simulink model "Simple_drive_model_current"  (R2017b)
settings: Solver=VariableStepAuto  StartTime=0.0  StopTime=5  RelTol=1e-3  EnableMultiTasking=on
values from neighbouring files (symbols this model uses):
  i = 120    [Drive_simple_variables.m]
  Jload = 5    [Drive_simple_variables.m]
  Jmotor = Jgear + Jrot    (= 0.003335)    [Drive_simple_variables.m]
  Kcur_Fdb = round(Uadc_inp*kadc/Imax)    [Drive_simple_variables.m]
  kcur_i = 1/Te    (= 139.830508475)    [Drive_simple_variables.m]
  kcur_p = Wcutoff_c*Te*Rrot/(Kpwc*Kcur_Fdb)    [Drive_simple_variables.m]
  Ke = Km    (= 1.41666666667)    [Drive_simple_variables.m]
  Km = Mrate/I    (= 1.41666666667)    [Drive_simple_variables.m]
  Kpos_Fdb = kps_int    (= 63661.9772368)    [Drive_simple_variables.m]
  kpos_p = Wcutoff_pos*Ts    [Drive_simple_variables.m]
  Kpwc = Un/Uc    (= 45)    [Drive_simple_variables.m]
  Kspd_Fdb = kps_int*Ts    (= 63.6619772368)    [Drive_simple_variables.m]
  kspd_i = 1/Tspd    [Drive_simple_variables.m]
  kspd_p = Wcutoff_s/ksn    [Drive_simple_variables.m]
  Lrot = 0.0059    [Drive_simple_variables.m]
  Rrot = 0.8250    (= 0.825)    [Drive_simple_variables.m]
  Tpwc = 0.00014    [Drive_simple_variables.m]
  Ts = 1e-3    (= 0.001)    [Drive_simple_variables.m]
undefined symbols (not defined in the file or in its folder): Ampl, Wsr
settings Model: Creator=Руслан  LastModifiedBy=Ruslan
settings OptimizationCC: LifeSpan=inf
settings DebuggingCC: SFUnexpectedBacktrackingDiag=warning  SFNoUnconditionalDefaultTransitionDiag=warning  SFExecutionAtInitializationDiag=none
settings CodeAppCC: StateflowObjectComments=on
settings GRTTargetCC: TargetLangStandard=C89/C90 (ANSI)  GeneratePreprocessorConditionals=Disable all
settings ConfigComp: CovMetricSettings=dw  CovHtmlReporting=on  CovSaveCumulativeToWorkspaceVar=on  CovSaveSingleToWorkspaceVar=on  CovExternalEMLEnable=off

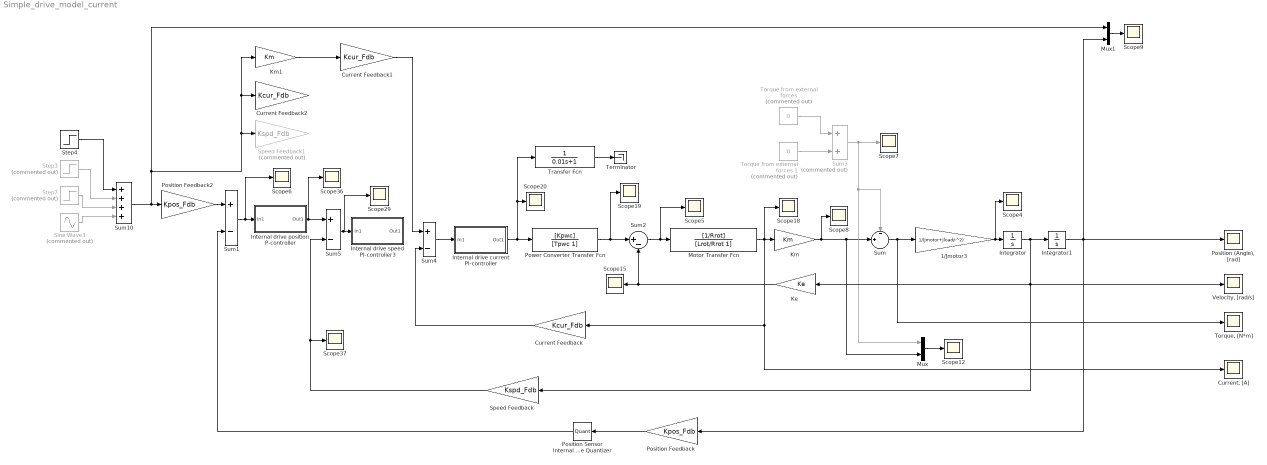
== system Simple_drive_model_current ==
  1/Jmotor3 : Gain  Gain=1/(Jmotor+Jload/i^2)  OutDataTypeStr=Inherit: Same as input  ParamDataTypeStr=Inherit: Same as input
  Current Feedback : Gain  Gain=Kcur_Fdb  OutDataTypeStr=Inherit: Same as input  ParamDataTypeStr=Inherit: Same as input
  Current Feedback1 : Gain  Gain=Kcur_Fdb  OutDataTypeStr=Inherit: Same as input  ParamDataTypeStr=Inherit: Same as input
  Current Feedback2 : Gain  Gain=Kcur_Fdb  OutDataTypeStr=Inherit: Same as input  ParamDataTypeStr=Inherit: Same as input
  "Current, [A]" : Scope
  Integrator : Integrator
  Integrator1 : Integrator
  Internal drive current PI-controller : Subsystem
  Internal drive position P-controller : Subsystem
  Internal drive speed PI-controller3 : Subsystem
  Ke : Gain  Gain=Ke  OutDataTypeStr=Inherit: Same as input  ParamDataTypeStr=Inherit: Same as input
  Km : Gain  Gain=Km  OutDataTypeStr=Inherit: Same as input  ParamDataTypeStr=Inherit: Same as input
  Km1 : Gain  Gain=Km  OutDataTypeStr=Inherit: Same as input  ParamDataTypeStr=Inherit: Same as input
  Motor Transfer Fcn : TransferFcn  Numerator=[1/Rrot]  Denominator=[Lrot/Rrot 1]
  Mux : Mux  Inputs=2
  Mux1 : Mux  Inputs=2
  "Position (Angle), [rad]" : Scope
  Position Feedback : Gain  Gain=Kpos_Fdb  OutDataTypeStr=Inherit: Same as input  ParamDataTypeStr=Inherit: Same as input
  Position Feedback2 : Gain  Gain=Kpos_Fdb  OutDataTypeStr=Inherit: Same as input  ParamDataTypeStr=Inherit: Same as input
  Position Sensor Internal Drive Quantizer : Quantizer  QuantizationInterval=1/Kpos_Fdb
  Power Converter Transfer Fcn : TransferFcn  Numerator=[Kpwc]  Denominator=[Tpwc 1]
  Scope{4..9,12,15,18..20,29,36..37} (14 alike) : Scope
  Sine Wave3 : Sin  Commented=on  Amplitude=Ampl  Frequency=Wsr  SampleTime=0
  Speed Feedback : Gain  Gain=Kspd_Fdb  OutDataTypeStr=Inherit: Same as input  ParamDataTypeStr=Inherit: Same as input
  Speed Feedback1 : Gain  Commented=on  Gain=Kspd_Fdb  OutDataTypeStr=Inherit: Same as input  ParamDataTypeStr=Inherit: Same as input
  Step3 : Step  Commented=on  Time=2  After=-1  SampleTime=0
  Step4 : Step  Time=0  SampleTime=0
  Step7 : Step  Commented=on  Time=2  SampleTime=0
  Sum : Sum  Inputs=-|+||
  Sum1 : Sum  Inputs=+-
  Sum10 : Sum  Inputs=4
  Sum2 : Sum  Inputs=|+-
  Sum3 : Sum  Commented=on  Inputs=2
  Sum4 : Sum  Inputs=+-
  Sum5 : Sum  Inputs=+-
  Terminator : Terminator
  "Torque from external forces " : Constant  Commented=on  Value=0
  Torque from external forces 1 : Constant  Commented=on  Value=0
  "Torque, [N*m]" : Scope
  Transfer Fcn : TransferFcn  Denominator=[0.01 1]
  "Velocity, [rad/s]" : Scope
  wires:
  Position Feedback/1 -> Position Sensor Internal Drive Quantizer/1
  Integrator1/1 -> Position Feedback/1, Mux1/2, "Position (Angle), [rad]"/1
  Sum4/1 -> Internal drive current PI-controller/1(In1)
  Sum5/1 -> Internal drive speed PI-controller3/1(In1), Scope29/1
  Speed Feedback/1 -> Scope37/1, Sum5/2
  Current Feedback/1 -> Sum4/2
  Sum1/1 -> Scope6/1, Internal drive position P-controller/1(In1)
  Km/1 -> Mux/2, Sum/2, Scope8/1
  Mux/1 -> Scope12/1
  Internal drive current PI-controller/1(Out1) -> Power Converter Transfer Fcn/1, Transfer Fcn/1, Scope20/1
  Power Converter Transfer Fcn/1 -> Scope19/1, Sum2/1
  Sum2/1 -> Scope5/1, Motor Transfer Fcn/1
  Sum/1 -> 1/Jmotor3/1, "Torque, [N*m]"/1
  1/Jmotor3/1 -> Scope4/1, Integrator/1
  Sum3/1 -> Sum/1, Mux/1, Scope7/1
  Motor Transfer Fcn/1 -> Km/1, Scope18/1, Current Feedback/1, "Current, [A]"/1
  Integrator/1 -> Integrator1/1, Speed Feedback/1, "Velocity, [rad/s]"/1, Ke/1
  Transfer Fcn/1 -> Terminator/1
  Step4/1 -> Sum10/1
  Step3/1 -> Sum10/2
  Step7/1 -> Sum10/3
  Position Feedback2/1 -> Sum1/1
  Mux1/1 -> Scope9/1
  Sum10/1 -> Position Feedback2/1, Mux1/1, Km1/1, Current Feedback2/1, Speed Feedback1/1
  Sine Wave3/1 -> Sum10/4
  Ke/1 -> Sum2/2, Scope15/1
  Position Sensor Internal Drive Quantizer/1 -> Sum1/2
  Internal drive position P-controller/1(Out1) -> Sum5/1, Scope36/1
  "Torque from external forces "/1 -> Sum3/1
  Torque from external forces 1/1 -> Sum3/2
  Km1/1 -> Current Feedback1/1
  Current Feedback1/1 -> Sum4/1

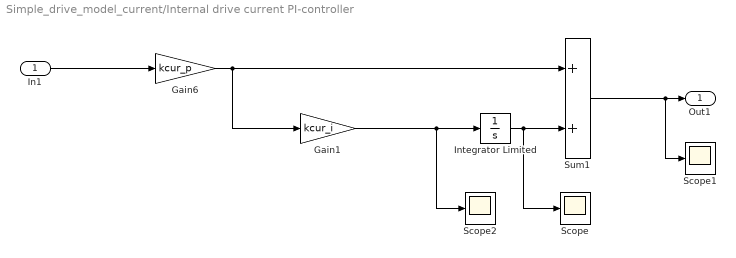
== system Simple_drive_model_current/Internal drive current PI-controller ==
  In1 : Inport
  Gain1 : Gain  Gain=kcur_i  OutDataTypeStr=Inherit: Same as input  ParamDataTypeStr=Inherit: Same as input
  Gain6 : Gain  Gain=kcur_p  OutDataTypeStr=Inherit: Same as input  ParamDataTypeStr=Inherit: Same as input
  Integrator Limited : Integrator  UpperSaturationLimit=0  LowerSaturationLimit=0
  Scope : Scope
  Scope1 : Scope
  Scope2 : Scope
  Sum1 : Sum
  Out1 : Outport
  wires:
  Gain1/1 -> Scope2/1, Integrator Limited/1
  Integrator Limited/1 -> Scope/1, Sum1/2
  Gain6/1 -> Gain1/1, Sum1/1
  In1/1 -> Gain6/1
  Sum1/1 -> Scope1/1, Out1/1

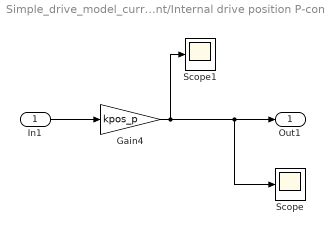
== system Simple_drive_model_current/Internal drive position P-controller ==
  In1 : Inport
  Gain4 : Gain  Gain=kpos_p  OutDataTypeStr=Inherit: Same as input  ParamDataTypeStr=Inherit: Same as input
  Scope : Scope
  Scope1 : Scope
  Out1 : Outport
  wires:
  In1/1 -> Gain4/1
  Gain4/1 -> Scope/1, Out1/1, Scope1/1

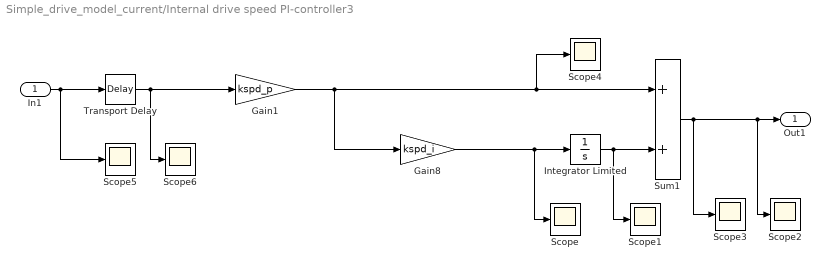
== system Simple_drive_model_current/Internal drive speed PI-controller3 ==
  In1 : Inport
  Gain1 : Gain  Gain=kspd_p  OutDataTypeStr=Inherit: Same as input  ParamDataTypeStr=Inherit: Same as input
  Gain8 : Gain  Gain=kspd_i  OutDataTypeStr=Inherit: Same as input  ParamDataTypeStr=Inherit: Same as input
  Integrator Limited : Integrator  UpperSaturationLimit=0  LowerSaturationLimit=0
  Scope{,1..6} (7 alike) : Scope
  Sum1 : Sum
  Transport Delay : TransportDelay  DelayTime=Ts
  Out1 : Outport
  wires:
  Gain8/1 -> Scope/1, Integrator Limited/1
  Integrator Limited/1 -> Scope1/1, Sum1/2
  Gain1/1 -> Gain8/1, Scope4/1, Sum1/1
  Sum1/1 -> Scope2/1, Out1/1, Scope3/1
  Transport Delay/1 -> Gain1/1, Scope6/1
  In1/1 -> Transport Delay/1, Scope5/1
